simulink model "Adaptive_and_Formation_control_main"  (R2020b)
settings: Solver=VariableStepAuto  StartTime=0.0  StopTime=160  RelTol=1e-3
libraries: mobileRoboticsLib x7, simulink x4, dsppolyfun x1
settings Model: Creator=user  LastModifiedBy=user

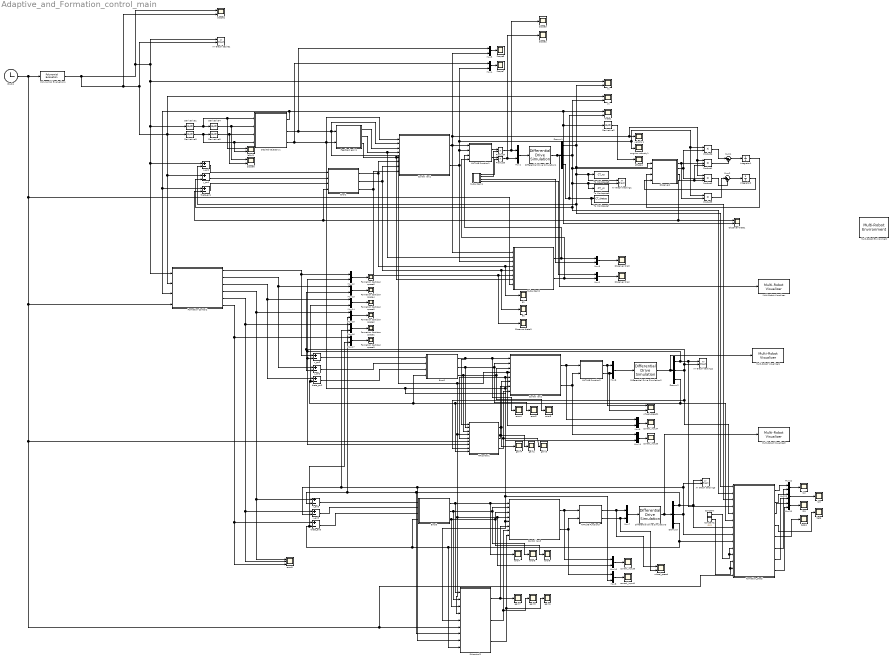
== system Adaptive_and_Formation_control_main ==
  Clock1 : Clock
  Constant : Constant  Value=1.5
  Constant1 : Constant  Value=pi/4
  Control law1 : MATLAB Function  TreatAsAtomicUnit=on
  Control law2 : MATLAB Function  TreatAsAtomicUnit=on
  Control law3 : MATLAB Function  TreatAsAtomicUnit=on
  Demux1 : Demux  Outputs=3
  Demux2 : Demux  Outputs=3
  Demux3 : Demux  Outputs=3
  Derivative{1..5} (5 alike) : Derivative  CoefficientInTFapproximation=0
  Desired trajectory1 : MATLAB Function  TreatAsAtomicUnit=on
  Differential Drive Simulation1 : mobileRoboticsLib/Kinematic Models/Differential Drive/Differential Drive Simulation  wheelRadius=0.075  wheelBase=0.3  initX=-0.15  initY=-0.13  initAngle=0  Ts=-1
      settings: SourceProductName=Mobile Robotics Simulation Toolbox
  Differential Drive Simulation2 : mobileRoboticsLib/Kinematic Models/Differential Drive/Differential Drive Simulation  wheelRadius=0.075  wheelBase=0.3  initX=-4  initY=-3  initAngle=pi+0.2  Ts=0.01
      settings: SourceProductName=Mobile Robotics Simulation Toolbox
  Differential Drive Simulation3 : mobileRoboticsLib/Kinematic Models/Differential Drive/Differential Drive Simulation  wheelRadius=0.075  wheelBase=0.3  initX=-3  initY=-0.5  initAngle=0.2  Ts=0.01
      settings: SourceProductName=Mobile Robotics Simulation Toolbox
  Error1 : MATLAB Function  TreatAsAtomicUnit=on
  Error2 : MATLAB Function  TreatAsAtomicUnit=on
  Error3 : MATLAB Function  TreatAsAtomicUnit=on
  Feedback gain1 : MATLAB Function  TreatAsAtomicUnit=on
  Formation Cartisian space{1..6} (6 alike) : Scope
  Formation Control2 : MATLAB Function  TreatAsAtomicUnit=on
  Integrator1 : Integrator  InitialCondition=800
  Integrator2 : Integrator  InitialCondition=200
  MATLAB Function1 : MATLAB Function  TreatAsAtomicUnit=on
  MATLAB Function2 : MATLAB Function  TreatAsAtomicUnit=on
  MATLAB Function3 : MATLAB Function  TreatAsAtomicUnit=on
  Multi-Robot Environment : mobileRoboticsLib/Environments/Multi-Robot Environment  numRobots=3  showWaypoints=off  showObjects=off  objectColors=[ 1, 0, 0; 0, 1, 0; 0, 0, 1 ]  objectMarkers='s'  showRobotIds=off  plotSensorLines=on
      settings: SourceProductName=Mobile Robotics Simulation Toolbox
  Multi-Robot Visualizer : mobileRoboticsLib/Environments/Multi-Robot Visualizer  idx=1  radius=0.03  robotColor=[0 0 1]  showTraj=on  hasLidar=off  sensorOffset=[0,0]  scanAngles=[-pi/4 0 pi/4]  maxNumScans=0  hasObjDetector=off  objDetectorOffset=[0,0]  objDetectorAngle=0  objDetectorFOV=pi/3  objDetectorMaxRange=5  hasRobotDetector=off  robotDetectorOffset=[0,0]  robotDetectorAngle=0  robotDetectorFOV=pi/3  robotDetectorMaxRange=5  robotDetectorNumDetections=0
      settings: SourceProductName=Mobile Robotics Simulation Toolbox
  Multi-Robot Visualizer1 : mobileRoboticsLib/Environments/Multi-Robot Visualizer  idx=2  radius=0.03  robotColor=[0 1 0]  showTraj=on  hasLidar=off  sensorOffset=[0,0]  scanAngles=[-pi/4 0 pi/4]  maxNumScans=0  hasObjDetector=off  objDetectorOffset=[0,0]  objDetectorAngle=0  objDetectorFOV=pi/3  objDetectorMaxRange=5  hasRobotDetector=off  robotDetectorOffset=[0,0]  robotDetectorAngle=0  robotDetectorFOV=pi/3  robotDetectorMaxRange=5  robotDetectorNumDetections=0
      settings: SourceProductName=Mobile Robotics Simulation Toolbox
  Multi-Robot Visualizer2 : mobileRoboticsLib/Environments/Multi-Robot Visualizer  idx=3  radius=0.03  robotColor=[1 0 0]  showTraj=on  hasLidar=off  sensorOffset=[0,0]  scanAngles=[-pi/4 0 pi/4]  maxNumScans=0  hasObjDetector=off  objDetectorOffset=[0,0]  objDetectorAngle=0  objDetectorFOV=pi/3  objDetectorMaxRange=5  hasRobotDetector=off  robotDetectorOffset=[0,0]  robotDetectorAngle=0  robotDetectorFOV=pi/3  robotDetectorMaxRange=5  robotDetectorNumDetections=0
      settings: SourceProductName=Mobile Robotics Simulation Toolbox
  Mux{1..17,20..22} (20 alike) : Mux  Inputs=2
  Observer slip2 : Scope
  Observer slip3 : Scope
  Observer theta1 : Scope  NumInputPorts=2
  Observer theta3 : Scope
  Observer1 : MATLAB Function  TreatAsAtomicUnit=on
  Polynomial Evaluation1 : dsppolyfun/Polynomial Evaluation  useConstCoeffs=on  constCoeffs=[0.05 0]
      settings: SourceProductBaseCode=DS
  Product1 : Product  Inputs=3
  Product2 : Product  Inputs=3
  Product{3..6} (4 alike) : Product
  RHcontrol1 : MATLAB Function  TreatAsAtomicUnit=on
  RHcontrol2 : MATLAB Function  TreatAsAtomicUnit=on
  Scope1 : Scope  NumInputPorts=2
  Scope{2..3,5,7} (4 alike) : Scope
  Scope6 : Scope  NumInputPorts=2
  Subsystem1 : Subsystem
  Subsystem2 : Subsystem
  Sum1 : Sum  Inputs=|--
  Sum2 : Sum  Inputs=|+-
  To Workspace7 : ToWorkspace  VariableName=CT_thetas  SampleTime=-1
      settings: Save2DSignal=2-D array (concatenate along first dimension)
  To Workspace8 : ToWorkspace  VariableName=CT_xs  SampleTime=-1
      settings: Save2DSignal=2-D array (concatenate along first dimension)
  To Workspace9 : ToWorkspace  VariableName=CT_ys  SampleTime=-1
      settings: Save2DSignal=2-D array (concatenate along first dimension)
  XY Graph desire1 : simulink/Sinks/XY Graph  xmin=-5  xmax=10  ymin=-5  ymax=10  st=-1
  XY Graph tracking1 : simulink/Sinks/XY Graph  xmin=-5  xmax=10  ymin=-5  ymax=10  st=-1
  XY Graph tracking2 : simulink/Sinks/XY Graph  xmin=-5  xmax=10  ymin=-5  ymax=10  st=-1
  XY Graph tracking3 : simulink/Sinks/XY Graph  xmin=-5  xmax=10  ymin=-5  ymax=10  st=-1
  angular velocity1 : Scope
  beta : Scope
  beta1 : Scope
  control_input{1,3..5} (4 alike) : Scope
  dtheta1 : Scope
  e1 : Scope
  e2 : Scope
  error{2,4..8} (6 alike) : Scope
  error9 : Scope  NumInputPorts=3
  formation_check : MATLAB Function  TreatAsAtomicUnit=on
  gain{2..7} (6 alike) : Scope
  l12 : Scope
  l13 : Scope
  l23 : Scope
  left d1 : Scope  NumInputPorts=2
  theta1 : Scope  NumInputPorts=2
  theta_err1 : Sum  Inputs=+-
  theta_err2 : Sum  Inputs=+-
  theta_err3 : Sum  Inputs=+-
  velocity1 : Scope
  wheel_speed : Scope  NumInputPorts=2
  wheel_speed1 : Scope  NumInputPorts=2
  x1 : Scope  NumInputPorts=2
  x_err1 : Sum  Inputs=+-
  x_err2 : Sum  Inputs=+-
  x_err3 : Sum  Inputs=+-
  y1 : Scope  NumInputPorts=2
  y_err1 : Sum  Inputs=+-
  y_err2 : Sum  Inputs=+-
  y_err3 : Sum  Inputs=+-
  wires:
  Error2/3(e3) -> error5/1, Control law2/3(et), RHcontrol1/3(et)
  RHcontrol1/1(k1) -> gain4/1, Control law2/6(k1)
  Control law1/1(v) -> MATLAB Function1/1(v), Product2/1, Product1/1, velocity1/1, Mux3/2, Subsystem2/1(v)  "v"
  Observer1/4(theta) -> Error1/4(theta), theta_err1/2, Observer theta1/1
  Derivative4/1 -> Scope6/1, Desired trajectory1/2(xd_dd)  "xd_dd"
  Polynomial Evaluation1/1 -> XY Graph desire1/2, Derivative3/1, y1/1, y_err1/1, Formation Control2/2(Ly), Scope1/2, Scope1/1, XY Graph desire1/1, x1/1, Derivative1/1, x_err1/1, Formation Control2/1(Lx)
  Subsystem1/2(il) -> Product4/2
  Mux3/1 -> Scope5/1
  Desired trajectory1/2(vd) -> Mux3/1, Mux9/2, Control law2/4(vd), Control law3/4(vd), Mux10/2, RHcontrol2/4(vd), RHcontrol1/4(vd), Feedback gain1/1(vd), Control law1/2(vd)  "vr"
  Sum2/1 -> Integrator2/1
  Product4/1 -> Scope3/1, Mux1/1
  Error1/3(e3) -> Control law1/8(e3), Observer theta3/1, Subsystem2/6(e3)  "e3"
  Subsystem2/1(Pl_hat) -> Mux5/1, MATLAB Function1/3(Pl_hat)
  Product6/1 -> Sum1/1
  Product2/1 -> Sum2/2
  Observer1/3(L) -> Product2/3, Product1/3
  Product5/1 -> Sum2/1
  Mux4/1 -> Scope7/1
  Observer1/2(z4_hat) -> Product2/2, Product6/2
  Observer1/1(z3_hat) -> Product5/2, Product1/2
  Control law2/1(v) -> Mux9/1, MATLAB Function2/1(v)  "v"
  Demux2/2 -> Mux13/2, y_err2/2, XY Graph tracking2/2, formation_check/5(x12), RHcontrol1/8(y)
  Control law2/2(w) -> MATLAB Function2/2(w), Mux11/1  "w"
  Differential Drive Simulation2/1 -> Multi-Robot Visualizer1/1, Demux2/1
  Demux3/2 -> XY Graph tracking3/2, RHcontrol2/8(y), Mux16/2, y_err3/2, formation_check/8(x22)
  Demux3/3 -> RHcontrol2/9(theta), Error3/4(theta), Mux17/2, theta_err3/2, formation_check/9(x23)
  Mux2/1 -> Observer slip2/1
  theta_err3/1 -> Error3/3(theta_error)
  x_err2/1 -> Error2/1(x_err)
  y_err2/1 -> Error2/2(y_err)
  Demux2/1 -> XY Graph tracking2/1, formation_check/4(x11), Mux12/2, RHcontrol1/7(x), x_err2/2
  Control law3/1(v) -> Mux10/1, MATLAB Function3/1(v)  "v"
  Error2/1(e1) -> RHcontrol1/1(ex), error4/1, Control law2/1(ex)
  Control law3/2(w) -> Mux8/1, MATLAB Function3/2(w)  "w"
  Differential Drive Simulation3/1 -> Multi-Robot Visualizer2/1, Demux3/1
  MATLAB Function3/2(wr) -> wheel_speed/2, Mux7/2
  Integrator1/1 -> Observer1/3(alpha)
  Mux5/1 -> Observer slip3/1
  Error3/1(e1) -> RHcontrol2/1(ex), error7/1, Control law3/1(ex)
  Subsystem1/3(pl) -> Mux5/2
  theta_err2/1 -> Error2/3(theta_error)
  RHcontrol1/3(k3) -> gain3/1, Control law2/8(k3)
  Mux6/1 -> Differential Drive Simulation2/1
  RHcontrol2/1(k1) -> gain7/1, Control law3/6(k1)
  Mux7/1 -> Differential Drive Simulation3/1
  Formation Control2/1(fx1) -> x_err2/1, Mux12/1
  Formation Control2/2(fy1) -> y_err2/1, Mux13/1
  Formation Control2/3(ft1) -> Mux14/1, theta_err2/1
  Clock1/1 -> Polynomial Evaluation1/1, Subsystem2/8(t), RHcontrol2/6(time), formation_check/14(times), RHcontrol1/6(time), Formation Control2/4(time)
  Demux1/2 -> To Workspace9/1, XY Graph tracking1/2, formation_check/2(l2), y_err1/2, Observer1/2(z2), y1/2
  MATLAB Function1/1(wl) -> Product4/1  "wl"
  Error2/2(e2) -> RHcontrol1/2(ey), error2/1, Control law2/2(ey)
  x_err1/1 -> Error1/1(x_err)
  MATLAB Function2/2(wr) -> wheel_speed1/2, Mux6/2  "wr"
  Subsystem1/1(ir) -> Product3/2
  Subsystem2/2(Pr_hat) -> MATLAB Function1/4(Pr_hat), Mux2/2
  theta_err1/1 -> Error1/3(theta_error)
  Derivative3/1 -> Desired trajectory1/4(yd_d), left d1/2, Derivative5/1  "yd_d"
  Formation Control2/6(fz2) -> Mux17/1, theta_err3/1, error9/3
  Control law1/2(w) -> Mux4/2, Product6/1, Product5/1, angular velocity1/1, MATLAB Function1/2(w), Subsystem2/3(w)  "w"
  y_err3/1 -> Error3/2(y_err)
  Derivative1/1 -> Derivative4/1, left d1/1, Desired trajectory1/1(xd_d)  "xd_d"
  MATLAB Function3/1(wl) -> wheel_speed/1, Mux7/1
  Integrator2/1 -> Observer1/4(beta)
  Demux1/3 -> formation_check/3(l3), To Workspace7/1, theta1/2
  Feedback gain1/2(k2) -> Subsystem2/2(k2), Control law1/4(k2)
  y_err1/1 -> Error1/2(y_err)
  Differential Drive Simulation1/1 -> Multi-Robot Visualizer/1, Demux1/1
  Feedback gain1/3(k3) -> Control law1/5(k3), Subsystem2/7(k3)
  Feedback gain1/1(k1) -> Control law1/3(k1)
  Desired trajectory1/1(td) -> theta_err1/1, Formation Control2/3(Lt), theta1/1, Observer theta1/2, Derivative2/1
  Error1/1(e1) -> e1/1, Subsystem2/4(e1), Control law1/6(e1)  "e1"
  Derivative5/1 -> Scope6/2, Desired trajectory1/3(yd_dd)  "yd_dd"
  Product3/1 -> Scope2/1, Mux1/2
  x_err3/1 -> Error3/1(x_err)
  Desired trajectory1/3(wd) -> RHcontrol2/5(wd), Control law3/5(wd), Mux8/2, Control law2/5(wd), RHcontrol1/5(wd), Mux11/2, Control law1/1(wd), Feedback gain1/2(wd), Mux4/1
  Error1/2(e2) -> e2/1, Subsystem2/5(e2), Control law1/7(e2)  "e2"
  Sum1/1 -> Integrator1/1
  Demux2/3 -> formation_check/6(x13), RHcontrol1/9(theta), Error2/4(theta), Mux14/2, theta_err2/2
  Demux3/1 -> XY Graph tracking3/1, formation_check/7(x21), RHcontrol2/7(x), Mux15/2, x_err3/2
  Mux1/1 -> Differential Drive Simulation1/1
  MATLAB Function2/1(wl) -> wheel_speed1/1, Mux6/1  "wl"
  Subsystem1/4(pr) -> Mux2/1
  RHcontrol1/2(k2) -> gain2/1, Control law2/7(k2)
  Demux1/1 -> formation_check/1(l1), x_err1/2, XY Graph tracking1/1, To Workspace8/1, Observer1/1(z1), x1/2
  MATLAB Function1/2(wr) -> Product3/1  "wr"
  Derivative2/1 -> dtheta1/1
  Product1/1 -> Sum1/2
  Formation Control2/4(fx2) -> Mux15/1, x_err3/1, error9/1
  Formation Control2/5(fy2) -> Mux16/1, y_err3/1, error9/2
  Mux11/1 -> control_input3/1
  Mux9/1 -> control_input4/1
  Mux12/1 -> Formation Cartisian space6/1
  Mux13/1 -> Formation Cartisian space4/1
  Mux14/1 -> Formation Cartisian space5/1
  Mux15/1 -> Formation Cartisian space2/1
  Mux17/1 -> Formation Cartisian space3/1
  Mux16/1 -> Formation Cartisian space1/1
  Error3/3(e3) -> error8/1, Control law3/3(et), RHcontrol2/3(et)
  Error3/2(e2) -> RHcontrol2/2(ey), error6/1, Control law3/2(ey)
  RHcontrol2/3(k3) -> Control law3/8(k3), gain6/1
  RHcontrol2/2(k2) -> Control law3/7(k2), gain5/1
  Mux8/1 -> control_input1/1
  Mux10/1 -> control_input5/1
  Constant/1 -> formation_check/11("d2 "), formation_check/10("d1 ")
  Constant1/1 -> formation_check/13(b2), formation_check/12(b1)
  formation_check/5(beta2) -> beta1/1
  formation_check/4(beta1) -> beta/1
  Mux20/1 -> l23/1
  formation_check/3(l13) -> Mux20/1
  formation_check/2(l23) -> Mux21/1
  Mux21/1 -> l13/1
  formation_check/1(l12) -> Mux22/1
  Mux22/1 -> l12/1
  formation_check/6(d1) -> Mux22/2
  formation_check/7(d2) -> Mux21/2
  formation_check/8(d3) -> Mux20/2

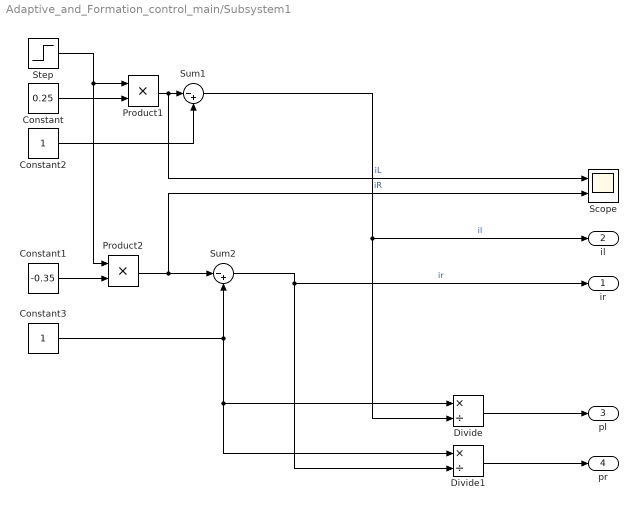
== system Adaptive_and_Formation_control_main/Subsystem1 ==
  Constant : Constant  Value=0.25
  Constant1 : Constant  Value=-0.35
  Constant2 : Constant
  Constant3 : Constant
  Divide : Product  Inputs=*/
  Divide1 : Product  Inputs=*/
  Product1 : Product
  Product2 : Product
  Scope : Scope  NumInputPorts=2
  Step : Step  Time=0  SampleTime=0
  Sum1 : Sum  Inputs=|-+
  Sum2 : Sum  Inputs=|-+
  ir : Outport
  il : Outport  Port=2
  pl : Outport  Port=3
  pr : Outport  Port=4
  wires:
  Sum1/1 -> Divide/2, il/1  "il"
  Step/1 -> Product2/1, Product1/1
  Constant3/1 -> Divide/1, Divide1/1, Sum2/2
  Product1/1 -> Scope/1, Sum1/1  "iL"
  Constant2/1 -> Sum1/2
  Sum2/1 -> ir/1, Divide1/2  "ir"
  Constant1/1 -> Product2/2
  Constant/1 -> Product1/2
  Product2/1 -> Scope/2, Sum2/1  "iR"
  Divide/1 -> pl/1
  Divide1/1 -> pr/1

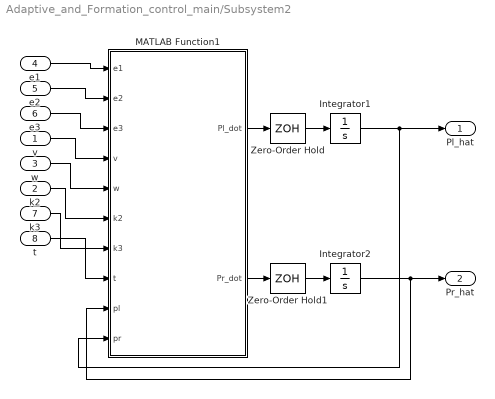
== system Adaptive_and_Formation_control_main/Subsystem2 ==
  v : Inport
  k2 : Inport  Port=2
  w : Inport  Port=3
  e1 : Inport  Port=4
  e2 : Inport  Port=5
  e3 : Inport  Port=6
  k3 : Inport  Port=7
  t : Inport  Port=8
  Integrator1 : Integrator  InitialCondition=1/0.85
  Integrator2 : Integrator  InitialCondition=1/1.2
  MATLAB Function1 : MATLAB Function  TreatAsAtomicUnit=on
  Zero-Order Hold : ZeroOrderHold  SampleTime=0.01
  Zero-Order Hold1 : ZeroOrderHold  SampleTime=0.01
  Pl_hat : Outport
  Pr_hat : Outport  Port=2
  wires:
  e2/1 -> MATLAB Function1/2(e2)
  Integrator1/1 -> Pl_hat/1, MATLAB Function1/10(pr)
  MATLAB Function1/2(Pr_dot) -> Zero-Order Hold1/1
  e3/1 -> MATLAB Function1/3(e3)
  w/1 -> MATLAB Function1/5(w)
  MATLAB Function1/1(Pl_dot) -> Zero-Order Hold/1
  k2/1 -> MATLAB Function1/6(k2)
  v/1 -> MATLAB Function1/4(v)
  e1/1 -> MATLAB Function1/1(e1)
  k3/1 -> MATLAB Function1/7(k3)
  Integrator2/1 -> Pr_hat/1, MATLAB Function1/9(pl)
  t/1 -> MATLAB Function1/8(t)
  Zero-Order Hold/1 -> Integrator1/1
  Zero-Order Hold1/1 -> Integrator2/1

== matlab function Adaptive_and_Formation_control_main/Error3 ==
  data: x_err input; e1 output; y_err input; theta_error input; theta input; e2 output; e3 output
function [e1,e2,e3] = error(x_err,y_err,theta_error,theta)
    e=[cos(theta) sin(theta) 0;-sin(theta) cos(theta) 0;0 0 1]*[x_err;y_err;theta_error];
    e1=e(1);
    e2=e(2);
    e3=e(3);
end

== matlab function Adaptive_and_Formation_control_main/Feedback gain1 ==
  data: k1 output; k2 output; k3 output; vd input; wd input
function [k1,k2,k3] = K(vd,wd)
    epsilon=1;
    kb=14;
    
    k1=2*epsilon*sqrt(wd^2+kb*vd^2);
    k3=k1;
    k2=kb*abs(vd);

end

== matlab function Adaptive_and_Formation_control_main/Formation Control2 ==
  data: Lx input; Ly input; fx1 output; Lt input; time input; fy1 output; ft1 output; fx2 output; fy2 output; fz2 output
function [fx1,fy1, ft1, fx2, fy2, fz2] = fcn(Lx,Ly,Lt,time)
    % Triangle Formation 
     if(time < 60)
        
        d = 1.5;
        theta1 = 3.14159/1.5;
        theta2 = 3.14159*3/2;
%         theta3 = ;
        %% First Robot SBOS
        fx1 = Lx + d * cos(Lt + theta1);
        fy1 = Ly + d * sin(Lt + theta1);
        ft1 = Lt;
        %% Second Robot SSOS
        d1 = 1.5;
        d2 = 1.5;
        dx = Lx - fx1;
        dy = Ly - fy1;
        M = (1/2) * (Lx * Lx - fx1 * fx1 + Ly * Ly - fy1 * fy1 - d1*d1 + d2*d2);
        a = 2 * (dx * dx + dy * dy); 
        b = 2 * (M * dx - dy* (dx * Ly - dy * Lx));
        c = (M - dy * Ly) * (M - dy * Ly) - (dy * Lx) * (dy * Lx) - (d1 * dy) * (d1 * dy);
        fx2 = (b + (b * b - 4 * a * c)) / a;
%         fx2 = (b - (b * b - 4 * a * c)) / a;
        fy2 = (M - dx * fx2) / dy;
        fz2 = Lt;
        
        
%         fx2 = Lx + d * cos(Lt + theta2);
%         fy2 = Ly + d * sin(Lt + theta2);
%         fz2 = Lt;
%         %% Third Robot
%         fx3 = Lx + d * cos(Lt + theta2);
%         fy3 = Ly + d * sin(Lt + theta2);
%         fz3 = Lt;

    %% My method of tracking two robot
        L = sqrt((Lx - fx1) * (Lx - fx1) + (Ly - fy1) * (Ly - fy1))
        k1 = (Ly - fy1) / (Lx - fx1);
        k2 = -1/k1;
        AE = (d1*d1 - d2*d2 + L*L)/(2*L);
        CE = d1 * d1 - AE * AE;
        x0 = Lx + AE / L * (fx1 - Lx);
        y0 = Ly + AE / L * (fy1 - Ly);
        fx2 = x0 - CE/sqrt(1+k2*k2); 
        fy2 = y0 + k2 * (fx2 - x0);
        fz2 = Lt;
    %Linear Formation
%     elseif(time >= 60 && time < 120)
%     
%         d = 0.15;
%         theta = 3.14159;
%         
%         fx1 = Lx + d * cos(Lt + theta);
%         fy1 = Ly + d * sin(Lt + theta);
%         ft1 = Lt;
%         fx2 = Lx + d * 2 * cos(Lt + theta);
%         fy2 = Ly + d * 2 * sin(Lt + theta);
%         fz2 = ft1;
%         
%     
%     % Closer Linear Formation
     else 
%     
         d = 0.3;
         theta = 3.14159;
               
         fx1 = Lx + d * cos(Lt + theta);
         fy1 = Ly + d * sin(Lt + theta);
         ft1 = Lt;
         fx2 = Lx + d * 2 * cos(Lt + theta);
         fy2 = Ly + d * 2 * sin(Lt + theta);
         fz2 = ft1;
    
        
     end


end

== matlab function Adaptive_and_Formation_control_main/MATLAB Function1 ==
  data: v input; wl output; w input; Pl_hat input; Pr_hat input; wr output
function [wl,wr] = IK(v,w,Pl_hat,Pr_hat)
    %parameters
    r=0.075;
    b=0.3;
    %inverse kinematics
%     wl = v/(r*il) - w*b/(r*il);
%     wr = v/(r*ir) + w*b/(r*ir);
    wl = v*Pl_hat/(r) - w*b*Pl_hat/(2*r);
    wr = v*Pr_hat/(r) + w*b*Pr_hat/(2*r);
end

== matlab function Adaptive_and_Formation_control_main/MATLAB Function2 ==
  data: v input; wl output; w input; wr output
function [wl,wr] = IK(v,w)
    %parameters
    r=0.075;
    b=0.3;
    %inverse kinematics
%     wl = v/(r*il) - w*b/(r*il);
%     wr = v/(r*ir) + w*b/(r*ir);
    wl = v/(r) - w*b/(2*r);
    wr = v/(r) + w*b/(2*r);
end

== matlab function Adaptive_and_Formation_control_main/MATLAB Function3 ==
  data: v input; wl output; w input; wr output
function [wl,wr] = IK(v,w)
    %parameters
    r=0.075;
    b=0.3;
    %inverse kinematics
%     wl = 0.1;
%     wr = 0.1;
    wl = v/(r) - w*b/(2*r);
    wr = v/(r) + w*b/(2*r);
end

== matlab function Adaptive_and_Formation_control_main/Observer1 ==
  data: z3_hat output; z4_hat output; z1 input; z2 input; alpha input; beta input; L output; theta output
function [z3_hat,z4_hat,L,theta] = K(z1,z2,alpha,beta)
    L = 100;
    z3_hat = alpha + L * z1;
    z4_hat = beta + L * z2;
    theta = atan2(z4_hat,z3_hat);
end

== matlab function Adaptive_and_Formation_control_main/RHcontrol2 ==
  data: ex input; ey input; et input; k1 output; k2 output; k3 output; vd input; wd input; time input; x input; y input; theta input
function [k1,k2,k3] = fcn(ex,ey,et, vd,wd,time,x,y,theta)
% SSOS
    ex_total = 0;
    ey_total = 0;
    et_total = 0;
    %% Select weiting matrix Q and matrix R 
    
    q1 = 0.01;
    q2 = 0.1;
    q3 = 0.5;
    R1 = 0;
    R2 = 0;
    R3 = 0;
    %% Formation control paramters
    d = 1.5;
    theta1 = 3.14159/1.5;
    theta2 = 3.14159*3/2;
    theta3 = 3.141593*1.25;
    
    %% Receding Horizon control
    Predict_horizon = 0.1;
    Sampling_time = 0.01;

    k3 = 0.35 + q3;
    k2 = 0.5 + vd * sin(et) / et;
    k1 = 0.5 + q1 + q2 * ey * ey / (ex * ex);
    
    for t = 0:Predict_horizon:Sampling_time
        if(time < 60)
            % Reference trajectory
    %         % First Robot SBOS
    %         fx1 = Lx + d * cos(Lt + theta1);
    %         fy1 = Ly + d * sin(Lt + theta1);
    %         ft1 = Lt;
            fx1 = 0.05*(t+time) + d * cos(theta1);
            fy1 = 0.05*(t+time) + d * sin(theta1);
            fz1 = 3.14159/4;
            % Second Robot SSOS
            d1 = 1.5;
            d2 = 1.5;
            dx = 0.05*(t+time) - fx1;
            dy = 0.05*(t+time) - fy1;
            M = (1/2) * (0.05*(t+time) * 0.05*(t+time) - fx1 * fx1 + 0.05*(t+time) * 0.05*(t+time) - fy1 * fy1 - d1*d1 + d2*d2);
            a = 2 * (dx * dx + dy * dy); 
            b = 2 * (M * dx - dy* (dx * 0.05*(t+time) - dy * 0.05*(t+time)));
            c = (M - dy * 0.05*(t+time)) * (M - dy * 0.05*(t+time)) - (dy * 0.05*(t+time)) * (dy * 0.05*(t+time)) - (d1 * dy) * (d1 * dy);
            fx2 = (b + (b * b - 4 * a * c)) / a;
    %         fx2 = (b - (b * b - 4 * a * c)) / a;
            fy2 = (M - dx * fx2) / dy;
            fz2 = 3.14159/4;
    %         fx2 = 0.05*(t+time) + d * cos(theta2);
    %         fy2 = 0.05*(t+time) + d * sin(theta2);
    %         fz2 = 3.14159/4;
    %         fx1 = Lx + d * cos(Lt + theta1);
    %         fy1 = Ly + d * sin(Lt + theta1);
    %         ft1 = Lt;
    %         
    %         dx = Lx - fx1;
    %         dy = Ly - fy1;
    %         M = (1/2) * ((Lx * Lx - fx1 * fx1) + (Ly * Ly - fy1 * fy1) - d*d + d*d);
    %         a = 2 * (dx * dx + dy * dy); 
    %         b = 2 * (M * dx - dy* (dx * Ly - dy * Lx));
    %         c = (M - dy * Ly) * (M - dy * Ly) - (dy * Lx) * (dy * Lx) - (d * dy) * (d * dy);
    %         fx2 = (b + sqrt((b * b - 4 * a * c))) / a;
    % %         fx2 = (b - (b * b - 4 * a * c)) / a;
    %         fy2 = (M - dx * fx2) / dy;
    %         fz2 = Lt;
        % My method of tracking two robot
            L = sqrt((0.05*(t+time) - fx1) * (0.05*(t+time) - fx1) + (0.05*(t+time) - fy1) * (0.05*(t+time) - fy1))
            k1 = (0.05*(t+time) - fy1) / (0.05*(t+time) - fx1);
            k2 = -1/k1;
            AE = (d1*d1 - d2*d2 + L*L)/(2*L);
            CE = d1 * d1 - AE * AE;
            x0 = 0.05*(t+time) + AE / L * (fx1 - 0.05*(t+time));
            y0 = 0.05*(t+time) + AE / L * (fy1 - 0.05*(t+time));
            fx2 = x0 - CE/sqrt(1+k2*k2); 
            fy2 = y0 + k2 * (fx2 - x0);
            fz2 = 3.14159/4;

        else % times > 20 (sec)
            d = 0.3
            fx2 = 0.05*(t+time) + 2 * d * cos(3.14159*1.25);
            fy2 = 0.05*(t+time) + 2 * d * sin(3.14159*1.25);
            fz2 = 3.14159/4;
        end
            % Optimal strategy LQR control 

        k3 = 0.35 + q3;
        if(et == 0)
            k2 = 0.5;
        else
            k2 = 0.5 + vd * sin(et) / et;
        end
        k1 = 0.5 + q1 + q2 * ey * ey / (ex * ex);

            % cauculate control input    

        if(et == 0)
            v = vd * cos(et) + k1 * ex;
            w = wd + k3 * et + k2 * vd * ey;
        else
            v = vd * cos(et) + k1 * ex;
            w = wd + k3 * et +  k2 * vd * ey * sin(et)/et;
        end

        % Forward kinematic   

        x = x + v * cos(theta) * Sampling_time;   
        y = y + v * sin(theta) * Sampling_time;
        theta = theta + w * Sampling_time;   
        
        % caculate next error
        e=[cos(theta) sin(theta) 0;-sin(theta) cos(theta) 0;0 0 1]*[x-fx2;y-fy2;theta-fz2];
        ex=e(1);
        ey=e(2);
        et=e(3);
        
        ex_total = ex_total + ex * Sampling_time;
        ey_total = ey_total + ey * Sampling_time;
        et_total = et_total + et * Sampling_time;
    end

    %% compute control gain
    
    k3 = 1 + q3;
    if(et_total == 0)
        k2 = 15;
    else
        k2 = 15 + 2 * vd * sin(et_total) / et_total;
    end
    
%     if(ey_total * ey_total / (ex_total * ex_total) <= 0.0000001)
%         k1 = 1 + q1 + q2 * ey_total * ey_total / (ex_total * ex_total);
%     else 
%         k1 = 2;
%     end
    
%     k1 = max(k1,5);
%     k2 = max(k2,100);
%     k3 = max(k3,5);
    
%     k1 = min(max(k1,5),10);
    k2 = min(max(k2,40),60);
    k3 = min(max(k3,1),2);
    
    if(ey_total * ey_total / (ex_total * ex_total) <= 2)
        k1 = 1 + q1 + q2 * ey_total * ey_total / (ex_total * ex_total);
    else 
        k1 = 2;
        k2 = 30;
        k3 = 3;
    end

 


end

== matlab function Adaptive_and_Formation_control_main/Subsystem2/MATLAB Function1 ==
  data: e1 input; Pl_dot output; e2 input; e3 input; v input; w input; Pr_dot output; k2 input; k3 input; t input; pl input; pr input
    function [Pl_dot,Pr_dot]  = observer(e1,e2,e3,v,w,k2,k3, t,pl, pr)
%% Paramaters
    gamma1 = 0.05;
    gamma2 = 0.05;
    r=0.075;
    b=0.3;
    k1 = 2;
    k2 = 10;
    k3 = 2;

        Pl_dot = gamma1 * (v - b*w/2) * (e1 * (e2/b + 1/2) - e1 * (e2 + k3 * e3)/b - k3 * (e2 + k3 * e3) / b - sin(e3)/(b*k2));
        Pr_dot = gamma2 * (v + b*w/2) * (-e1 * (e2/b - 1/2) + e1 * (e2 + k3 * e3)/b + k3 * (e2 + k3 * e3) / b + sin(e3)/(b*k2));
%%
%     %parameters
%     r=0.075;
%     b=0.3;
%     p1=5;
%     p2=5;
% 
%     if (t<0.1)
%         iLdot=1;
%         iRdot=1;
%     else
%         iLdot=p1*((e2/b + 1/2)*e1*v - (e2/2 + b/4)*e1*w - sin(e3)/k2*(v/b - w/2));
%         iRdot=p2*(-(e2/b - 1/2)*e1*v - (e2/2 - b/4)*e1*w + sin(e3)/k2*(v/b + w/2));
% 
%     end


end

== matlab function Adaptive_and_Formation_control_main/RHcontrol1 ==
  data: ex input; ey input; et input; k1 output; k2 output; k3 output; vd input; wd input; time input; x input; y input; theta input
function [k1,k2,k3] = fcn(ex,ey,et, vd,wd,time,x,y,theta)
    ex_total = 0;
    ey_total = 0;
    et_total = 0;
    %% Select weiting matrix Q and matrix R 
    
    q1 = 0.02;
    q2 = 0.02;
    q3 = 0.015;
    R1 = 0;
    R2 = 0;
    R3 = 0;
    
    %% Formation control paramters
    d = 1.5;
    theta1 = 3.14159/1.5;
    theta2 = 3.14159*3/2;
    
    %% Receding Horizon control
    Predict_horizon = 0.1;
    Sampling_time = 0.01;

    k3 = 0.35 + q3;
    k2 = 0.5 + vd * sin(et) / et;
    k1 = 0.5 + q1 + q2 * ey * ey / (ex * ex);
    
    for t = 0:Predict_horizon:Sampling_time
        
        % Reference trajectory
        if (time < 60)
            fx1 = 0.05*(t+time) + d * cos(theta1);
            fy1 = 0.05*(t+time) + d * sin(theta1);
            fz1 = 3.14159/4;
        else % times > 20 (sec)
            d = 0.3
            fx1 = 0.05*(t+time) + d * cos(3.14159*1.25);
            fy1 = 0.05*(t+time) + d * sin(3.14159*1.25);
            fz1 = 3.14159/4;
        end
        % Optimal strategy LQR control 
    
        k3 = 0.35 + q3;
        if(et == 0)
            k2 = 0.5;
        else
            k2 = 0.5 + vd * sin(et) / et;
        end
        k1 = 0.5 + q1 + q2 * ey * ey / (ex * ex);
        
        % caculate control input    
    
        if(et == 0)
            v = vd * cos(et) + k1 * ex;
            w = wd + k3 * et + k2 * vd * ey;
        else
            v = vd * cos(et) + k1 * ex;
            w = wd + k3 * et +  k2 * vd * ey * sin(et)/et;
        end
        
        % Forward kinematic   
        
        x = x + v * cos(theta) * Sampling_time;   
        y = y + v * sin(theta) * Sampling_time;
        theta = theta + w * Sampling_time;   
        
        % caculate next error
        ex_total = ex_total + ex * Sampling_time;
        ey_total = ey_total + ey * Sampling_time;
        et_total = et_total + et * Sampling_time;
        
        
        e=[cos(theta) sin(theta) 0;-sin(theta) cos(theta) 0;0 0 1]*[x-fx1;y-fy1;theta-fz1];
        ex=e(1);
        ey=e(2);
        et=e(3);
    end

    %% compute control gain
    k3 = 1 + q3;
    if(et_total == 0)
        k2 = 15;
    else
        k2 = 15 + 2 * vd * sin(et_total) / et_total;
    end
    

    
%     k1 = max(k1,5);
%     k2 = max(k2,100);
%     k3 = max(k3,5);
    
%     k1 = min(max(k1,5),10);
    k2 = min(max(k2,2),40);
    k3 = min(max(k3,1),2);
    

    if(ey_total * ey_total / (ex_total * ex_total) <= 30)
        k1 = 1 + q1 + q2 * ey_total * ey_total / (ex_total * ex_total);
    else 
        k1 = 2;
        k2 = 10;
        k3 = 3;
    end
 


end

== matlab function Adaptive_and_Formation_control_main/formation_check ==
  data: l1 input; l12 output; l2 input; l23 output; l3 input; x11 input; x12 input; x13 input; x21 input; x22 input; x23 input; d1 input; d2 input; b1 input; b2 input; l13 output; beta1 output; beta2 output; d1 output; d2 output; times input; d3 output
function [l12,l23,l13,beta1,beta2,d1, d2,d3] = IK(l1,l2,l3,x11,x12,x13,x21,x22,x23,d1,d2, b1,b2,times)
    
    if(times < 60)
        l12 = sqrt((l1 - x11) * (l1 - x11) + (l2 - x12) * (l2 - x12));
        l23 = sqrt((l1 - x21) * (l1 - x21) + (l2 - x22) * (l2 - x22));
        l13 = sqrt((x21 - x11) * (x21 - x11) + (x22 - x12) * (x22 - x12));
        d2 = 1.85
        d3 = 1.85
        beta1 = b1 - x13;
        beta2 = b2 - x23;
    else
        l12 = sqrt((l1 - x11) * (l1 - x11) + (l2 - x12) * (l2 - x12));
        l23 = sqrt((l1 - x21) * (l1 - x21) + (l2 - x22) * (l2 - x22));
        l13 = sqrt((x21 - x11) * (x21 - x11) + (x22 - x12) * (x22 - x12));
        d1 = 0.3;
        d2 = 0.6;
        d3 = 0.3;
        beta1 = 3.14159/4 - x13;
        beta2 = 3.14159/4 - x23;
    end
end

== matlab function Adaptive_and_Formation_control_main/Control law1 ==
  data: wd input; vd input; v output; k1 input; k2 input; k3 input; e1 input; e2 input; e3 input; w output
function [v,w] = fcn(wd,vd,k1,k2,k3,e1,e2,e3)
    v=zeros(1);
    w=zeros(1);
    vmax=0.15;
    wmax=0.45;
    
    
%    vc=vd*cos(e3)+k1*e1;
%    wc=wd+k2*sign(vd)*e2+k3*e3;
    
    %% gain 
    
    k11 = 2;
    k22 = 10;
    k33 = 2;
    
    %%
    wc = wd + vd / 2 * (k22 * (e2 + k33 * e3) + sin(e3) / k33); 
    vc = vd * cos(e3) + k33 * e3 * wc + k11 * e1;
%     wc=wd+k2*(vd)*e2+k3*sin(e3);

    sigma=max([abs(vc/vmax),abs(wc/wmax),1]);
    if(sigma==1)
        v=vc;
        w=wc;
    elseif(sigma==vc/vmax)
        v=sign(vc)*vmax;
        w=wc/sigma;
    else
        v=vc/sigma;
        w=sign(wc)*wmax;

    end
end

== matlab function Adaptive_and_Formation_control_main/Control law2 ==
  data: ex input; ey input; v output; et input; vd input; wd input; w output; k1 input; k2 input; k3 input
function [v,w] = fcn(ex,ey,et,vd,wd,k1,k2,k3)
%     q1 = 5;
%     q2 = 10;
%     q3 = 5;
%     k3 = 3.5 + q3;
%     k2 = 5 + vd * sin(et) / et;
%     k1 = 5 + q1 + q2 * ey * ey / (ex * ex);
%     
%     
%     k1 = max(k1,5);
%     k2 = max(k2,5);
%     k3 = max(k3,2.5);
%     
%     k1 = min(k1,20);
%     k2 = min(k2,20);
%     k3 = min(k3,20);
%     ratio = 0.5;
%     vd = vd * ratio;
%     wd = wd * ratio;
    if(et == 0)
        v = vd * cos(et) + k1 * ex;
        w = wd + k3 * et + k2 * vd * ey;
    else
        v = vd * cos(et) + k1 * ex;
        w = wd + k3 * et +  k2 * vd * ey * sin(et)/et;
    end

end

== matlab function Adaptive_and_Formation_control_main/Control law3 ==
  data: ex input; ey input; v output; et input; vd input; wd input; w output; k1 input; k2 input; k3 input
function [v,w] = fcn(ex,ey,et,vd,wd,k1,k2,k3)
%     q1 = 5;
%     q2 = 10;
%     q3 = 5;
%     k3 = 3.5 + q3;
%     k2 = 5 + vd * sin(et) / et;
%     k1 = 5 + q1 + q2 * ey * ey / (ex * ex);
%     
%     
%     k1 = max(k1,5);
%     k2 = max(k2,5);
%     k3 = max(k3,2.5);
%     
%     k1 = min(k1,20);
%     k2 = min(k2,20);
%     k3 = min(k3,20);
%     ratio = 0.5;
%     vd = vd * ratio;
%     wd = wd * ratio;
    if(et == 0)
        v = vd * cos(et) + k1 * ex;
        w = wd + k3 * et + k2 * vd * ey;
    else
        v = vd * cos(et) + k1 * ex;
        w = wd + k3 * et +  k2 * vd * ey * sin(et)/et;
    end

end

== matlab function Adaptive_and_Formation_control_main/Desired trajectory1 ==
  data: xd_d input; td output; xd_dd input; yd_dd input; yd_d input; vd output; wd output
function [td,vd,wd] = cmd_generation(xd_d,xd_dd,yd_dd,yd_d)
%    if atan2(yd_d,xd_d)<0
%        td=atan2(yd_d,xd_d)+2*pi;
%    else
        td=atan2(yd_d,xd_d);
%    end
    vd = sqrt(xd_d^2+yd_d^2);
    if(xd_d^2+yd_d^2==0)
        wd=0;
    else
        wd=(yd_dd*xd_d-xd_dd*yd_d)/(xd_d^2+yd_d^2);
    end
end

== matlab function Adaptive_and_Formation_control_main/Error1 ==
  data: x_err input; e1 output; y_err input; theta_error input; theta input; e2 output; e3 output
function [e1,e2,e3] = error(x_err,y_err,theta_error,theta)
    e=[cos(theta) sin(theta) 0;-sin(theta) cos(theta) 0;0 0 1]*[x_err;y_err;theta_error];
    e1=e(1);
    e2=e(2);
    e3=e(3);
end

== matlab function Adaptive_and_Formation_control_main/Error2 ==
  data: x_err input; e1 output; y_err input; theta_error input; theta input; e2 output; e3 output
function [e1,e2,e3] = error(x_err,y_err,theta_error,theta)
    e=[cos(theta) sin(theta) 0;-sin(theta) cos(theta) 0;0 0 1]*[x_err;y_err;theta_error];
    e1=e(1);
    e2=e(2);
    e3=e(3);
end
